simulink model "HydrolicTankSystem"  (R2021a)
settings: Solver=FixedStepAuto  StartTime=0.0  StopTime=60  FixedStep=10e-5  RelTol=1e-3
settings Model: Creator=kadir  LastModifiedBy=kadir

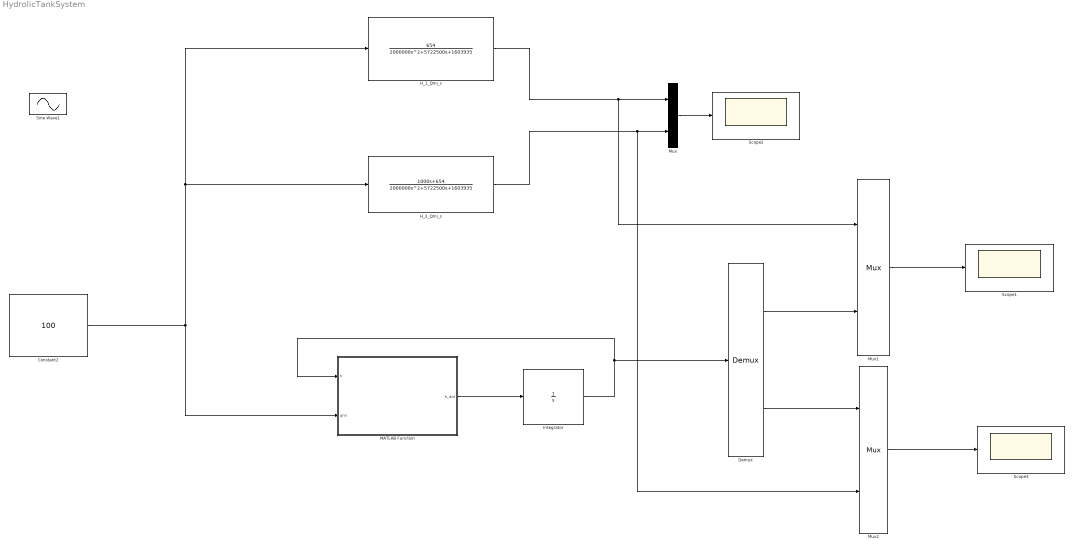
== system HydrolicTankSystem ==
  Constant2 : Constant  Value=100
  Demux : Demux  Outputs=2
  H_1_Qmi_s : TransferFcn  Numerator=[654]  Denominator=[2000000 5722500 1603935]
  H_2_Qmi_s : TransferFcn  Numerator=[1000 654]  Denominator=[2000000 5722500 1603935]
  Integrator : Integrator  InitialCondition=[2;1]
  MATLAB Function : MATLAB Function  TreatAsAtomicUnit=on
  Mux : Mux  Inputs=2
  Mux1 : Mux  Inputs=2
  Mux2 : Mux  Inputs=2
  Scope1 : Scope
  Scope2 : Scope
  Scope3 : Scope
  Sine Wave1 : Sin  Amplitude=5  Bias=5  Frequency=2*pi*0.1  SampleTime=0
  wires:
  H_1_Qmi_s/1 -> Mux1/1, Mux/1
  H_2_Qmi_s/1 -> Mux2/2, Mux/2
  Mux/1 -> Scope2/1
  MATLAB Function/1(h_dot) -> Integrator/1
  Integrator/1 -> MATLAB Function/1(h), Demux/1
  Constant2/1 -> H_1_Qmi_s/1, H_2_Qmi_s/1, MATLAB Function/2(qmi)
  Demux/1 -> Mux1/2
  Mux1/1 -> Scope1/1
  Demux/2 -> Mux2/1
  Mux2/1 -> Scope3/1

== matlab function HydrolicTankSystem/MATLAB Function ==
  data: h input; h_dot output; qmi input
function h_dot = fcn(h,qmi)

%%
ro = 1000;
A1 = 3;
A2 = 2;
R1 = 5;
R2 = 4;
g = 9.81;


A = [-g/(R1*A1), g/(R1*A1);g/(R1*A2), (-g/(R1*A2) + (-g/(R2*A2)))];

B = [0;1/(ro*A2)];

h_dot = A*h + B*qmi;

end
